simulink model "CRAB_TRACK"  (R2019b)
settings: Solver=VariableStepAuto  StartTime=0.0  StopTime=inf  RelTol=1e-3
undefined symbols (not defined in the file): Horn, magnitude, none, Rec, Schunck, SDTV, strel, videoinput
libraries: simulink x8, visionanalysis x3, visionconversions x2, visionstatistics x2, visionmorphops x2, dspsigattribs x2, dspindex x2, raspberrypilib x2, visiontextngfix x2, dspstat3 x2, imaqlib x1, dspmtrx3 x1
settings Model: Creator=danie  LastModifiedBy=danie

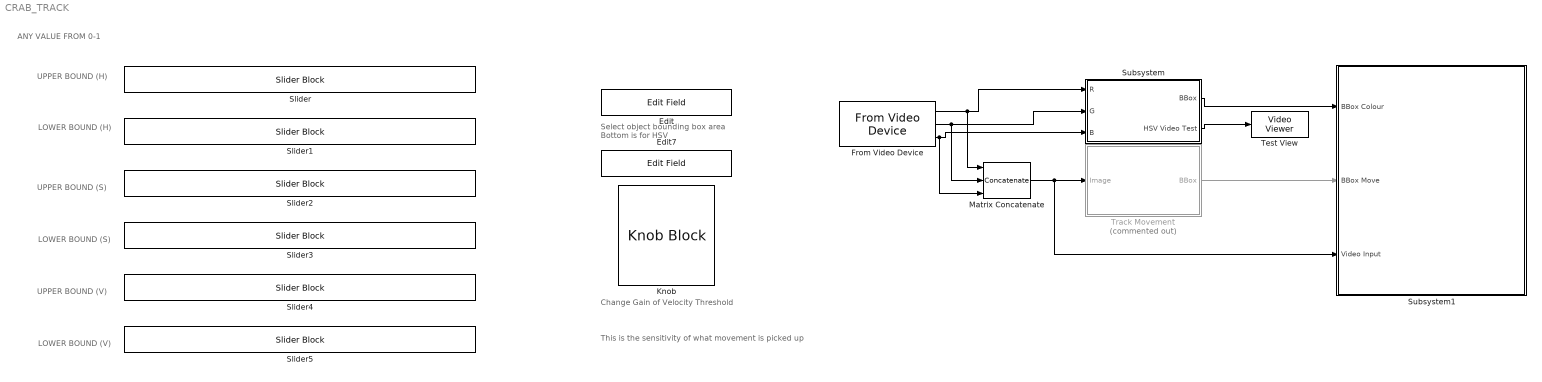
== system CRAB_TRACK ==
  note: ANY VALUE FROM 0-1
  note: LOWER BOUND (H)
  note: UPPER BOUND (H)
  note: This is the sensitivity of what movement is picked up
  note: Change Gain of Velocity Threshold
  note: Select object bounding box area
      | Bottom is for HSV
  note: UPPER BOUND (S)
  note: UPPER BOUND (V)
  note: LOWER BOUND (S)
  note: LOWER BOUND (V)
  Edit : EditField  LabelPosition=Hide  ShowInitialText=on  Alignment=Center
  Edit7 : EditField  LabelPosition=Hide  ShowInitialText=on  Alignment=Center
  From Video Device : imaqlib/From Video Device  DeviceMenu=winvideo 1 (USB_Camera)  Device=winvideo 1 (USB_Camera)  ObjConstructor=videoinput('winvideo', 1)  VideoFormatMenu=MJPG_1920x1080  VideoFormat=MJPG_1920x1080  VideoSource=input1  ROIPosition=[0 0 1080 1920]  EnableHWTrigger=off  TriggerConfiguration=none/none  SampleTime=1/30  OutputPortsMode=Separate color signals  DataType=single  CanDoHWTrigger=no  ReturnedColorSpace=rgb  BlockHandle=5428.0005  ROIWidth=1920  ROIHeight=1080  ROIColumn=0  ROIRow=0  EngXMLPath=E:\Matlab\toolbox\imaq\imaq\private  DevXMLPath=C:\ProgramData\MATLAB\SupportPackages\R2019b\toolbox\imaq\supportpackages\genericvideo\adaptor\win64  EngLibPath=E:\Matlab\toolbox\imaq\imaqblks\imaqmex\win64  ColorSpace=rgb  BayerSensorAlignment=grbg  ImaqMode=off
      settings: SourceProductName=Image Acquisition Toolbox
  Knob : KnobBlock
  Matrix Concatenate : Concatenate  NumInputs=3  Mode=Multidimensional array  ConcatenateDimension=3
  Slider{,1..5} (6 alike) : SliderBlock  ScaleMax=1
  Subsystem : Subsystem
  Subsystem1 : Subsystem
  Test View : VideoViewer  FigPos=[962 1037 958 929]
  Track Movement : Subsystem  Commented=on
  wires:
  From Video Device/1 -> Matrix Concatenate/1, Subsystem/1(R)
  Track Movement/1(BBox) -> Subsystem1/2(BBox Move)
  Subsystem/1(BBox) -> Subsystem1/1(BBox Colour)
  Subsystem/2(HSV Video Test) -> Test View/1
  From Video Device/2 -> Matrix Concatenate/2, Subsystem/2(G)
  From Video Device/3 -> Matrix Concatenate/3, Subsystem/3(B)
  Matrix Concatenate/1 -> Subsystem1/3(Video Input), Track Movement/1(Image)

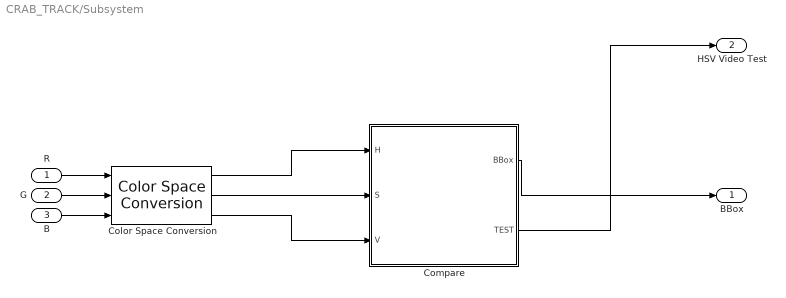
== system CRAB_TRACK/Subsystem ==
  R : Inport
  G : Inport  Port=2
  B : Inport  Port=3
  Color Space Conversion : visionconversions/Color Space  Conversion  conversion=Obsolete  conversionActive=R'G'B' to HSV  wp_str=D65  rec=Rec. 601 (SDTV)  sys=1125/60/2:1  imagePorts=Separate color signals
  Compare : Subsystem
  BBox : Outport
  HSV Video Test : Outport  Port=2
  wires:
  Compare/1(BBox) -> BBox/1
  Compare/2(TEST) -> HSV Video Test/1
  R/1 -> Color Space Conversion/1
  G/1 -> Color Space Conversion/2
  B/1 -> Color Space Conversion/3
  Color Space Conversion/1 -> Compare/1(H)
  Color Space Conversion/2 -> Compare/2(S)
  Color Space Conversion/3 -> Compare/3(V)

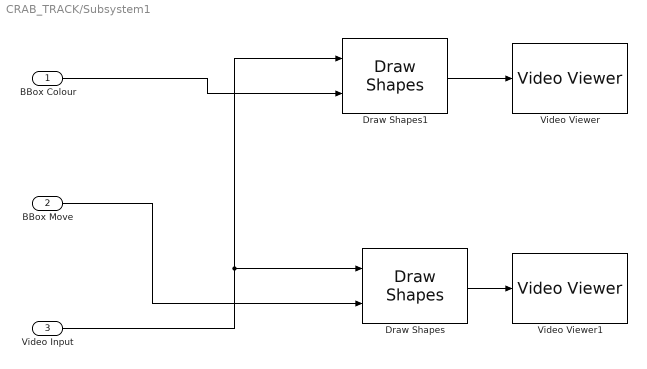
== system CRAB_TRACK/Subsystem1 ==
  BBox Colour : Inport
  BBox Move : Inport  Port=2
  Video Input : Inport  Port=3
  Draw Shapes : visiontextngfix/Draw Shapes  shape=Rectangles  fill=off  lineWidth=1  fillClrSource=Specify via dialog  display=User-specified value  intensity=200  color=[0 255 0]  opacity=0.6  viewport=Entire image  antialiasing=off  inType=Obsolete  imagePorts=One multidimensional signal  roundingMode=Floor  overflowMode=off  memoryMode=Specify word length  memoryWordLength=16  prodOutputMode=Binary point scaling  prodOutputWordLength=32  prodOutputFracLength=14  prodOutputSlope=2^-14  accumSlope=2^-14  memoryFracLength=15
      settings: SourceProductName=Computer Vision Toolbox
  Draw Shapes1 : visiontextngfix/Draw Shapes  shape=Rectangles  fill=off  lineWidth=1  fillClrSource=Specify via dialog  display=User-specified value  intensity=200  color=[0 255 0]  opacity=0.6  viewport=Entire image  antialiasing=off  inType=Obsolete  imagePorts=One multidimensional signal  roundingMode=Floor  overflowMode=off  memoryMode=Specify word length  memoryWordLength=16  prodOutputMode=Binary point scaling  prodOutputWordLength=32  prodOutputFracLength=14  prodOutputSlope=2^-14  accumSlope=2^-14  memoryFracLength=15
      settings: SourceProductName=Computer Vision Toolbox
  Video Viewer : VideoViewer  FigPos=[962 1037 958 929]
  Video Viewer1 : VideoViewer  FigPos=[2 517 958 409]
  wires:
  Draw Shapes/1 -> Video Viewer1/1
  Video Input/1 -> Draw Shapes1/1, Draw Shapes/1
  BBox Move/1 -> Draw Shapes/2
  Draw Shapes1/1 -> Video Viewer/1
  BBox Colour/1 -> Draw Shapes1/2

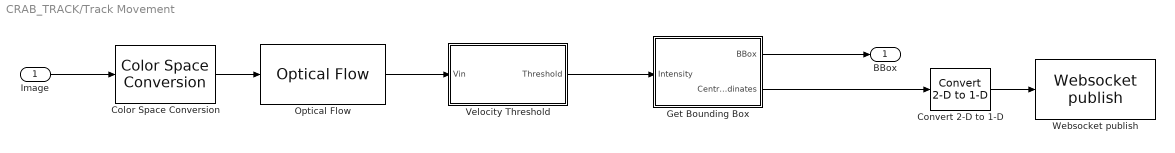
== system CRAB_TRACK/Track Movement ==
  Image : Inport
  Color Space Conversion : visionconversions/Color Space  Conversion  conversion=Obsolete  conversionActive=R'G'B' to intensity  wp_str=D65  rec=Rec. 601 (SDTV)  sys=1125/60/2:1  imagePorts=One multidimensional signal
  Convert 2-D to 1-D : dspsigattribs/Convert 2-D to 1-D
      settings: SourceProductName=DSP System Toolbox  SourceProductBaseCode=DS
  Get Bounding Box : Subsystem
  Optical Flow : visionanalysis/Optical Flow  method=Horn-Schunck  gradMethod=Difference filter [-1 1]  which2img=Current frame and N-th frame back  N=1  lambda=1  numInports=3  sigmaS=1.5  sigmaW=1  discardNormalFlow=off  outputCurrentImage=off  stop_criteria=When maximum number of iterations is reached  maxIter=10  maxAllowAbsDiff=eps  outVelForm=Horizontal and vertical components in complex form  eigTh=0.0039  roundingMode=Nearest  overflowMode=on  prodOutputMode=Binary point scaling  prodOutputWordLength=32  prodOutputFracLength=20  prodOutputSlope=2^-20  accumSlope=2^-20  memorySlope=2^-20  firstCoeffSlope=2^-20  outputMode=Binary point scaling  outputWordLength=32  outputFracLength=20  outputSlope=2^-20
      settings: SourceProductName=Computer Vision Toolbox  SourceProductBaseCode=VP
  Velocity Threshold : Subsystem
  Websocket publish : raspberrypilib/Websocket publish  UniqueBlockID=webPub 1  IPAddress=127.0.0.1  Port=9000  NumberOfSignals=1
      settings: SourceProductName=Simulink Support Package for Raspberry Pi Hardware  SourceProductBaseCode=RASPPI
  BBox : Outport
  wires:
  Image/1 -> Color Space Conversion/1
  Optical Flow/1 -> Velocity Threshold/1(Vin)
  Color Space Conversion/1 -> Optical Flow/1
  Velocity Threshold/1(Threshold) -> Get Bounding Box/1(Intensity)
  Get Bounding Box/2(Central Coordinates) -> Convert 2-D to 1-D/1
  Get Bounding Box/1(BBox) -> BBox/1
  Convert 2-D to 1-D/1 -> Websocket publish/1

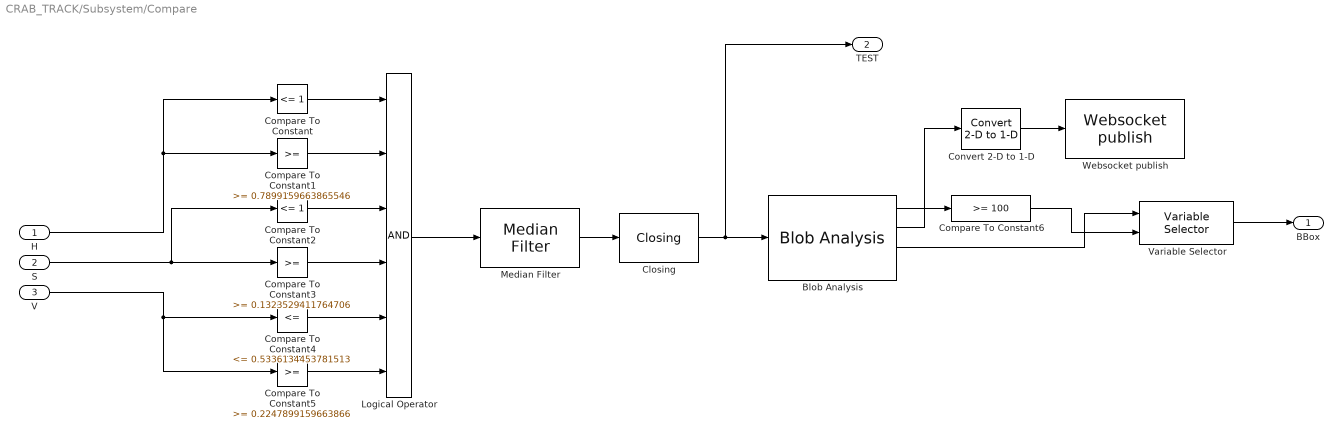
== system CRAB_TRACK/Subsystem/Compare ==
  H : Inport
  S : Inport  Port=2
  V : Inport  Port=3
  Blob Analysis : visionstatistics/Blob Analysis  Tag=vipblks_row_conv  area=on  centroid=on  bBox=on  majorAxis=off  minorAxis=off  angle=off  eccentricity=off  equivDiameterSq=off  extent=off  perimeter=off  outDT=double  conn=8  isLabel=on  maxBlobs=50  warnIfNumBlobsExceeded=on  isCount=off  useMinArea=off  minArea=0  useMaxArea=off  maxArea=intmax('uint32')  excludeBorderBlob=off  isOutVarDim=off  isFill=on  fillValues=-1  roundingMode=Floor  overflowMode=off  prodOutputMode=Binary point scaling  prodOutputWordLength=32  prodOutputFracLength=16  prodOutputSlope=2^-16  accumMode=Binary point scaling  accumWordLength=32  accumFracLength=0  accumSlope=2^0  outputMode=Binary point scaling  outputWordLength=32  outputFracLength=16  outputSlope=2^-16  memorySlope=2^-16  firstCoeffMode=Binary point scaling  firstCoeffWordLength=16  firstCoeffFracLength=14  firstCoeffSlope=2^-14  secondCoeffMode=Binary point scaling  secondCoeffWordLength=32  secondCoeffFracLength=16  secondCoeffSlope=2^-16
      settings: SourceProductName=Computer Vision Toolbox
  Closing : visionmorphops/Closing  nhoodsrc=Specify via dialog  strel=strel('line',5,45)
      settings: SourceProductName=Computer Vision Toolbox  SourceProductBaseCode=VP
  Compare To Constant : simulink/Logic and Bit Operations/Compare To Constant  relop=<=  const=1  OutDataTypeStr=boolean
  Compare To Constant1 : simulink/Logic and Bit Operations/Compare To Constant  relop=>=  const=0.7899159663865546  OutDataTypeStr=boolean
  Compare To Constant2 : simulink/Logic and Bit Operations/Compare To Constant  relop=<=  const=1  OutDataTypeStr=boolean
  Compare To Constant3 : simulink/Logic and Bit Operations/Compare To Constant  relop=>=  const=0.1323529411764706  OutDataTypeStr=boolean
  Compare To Constant4 : simulink/Logic and Bit Operations/Compare To Constant  relop=<=  const=0.5336134453781513  OutDataTypeStr=boolean
  Compare To Constant5 : simulink/Logic and Bit Operations/Compare To Constant  relop=>=  const=0.2247899159663866  OutDataTypeStr=boolean
  Compare To Constant6 : simulink/Logic and Bit Operations/Compare To Constant  relop=>=  const=100  OutDataTypeStr=boolean
  Convert 2-D to 1-D : dspsigattribs/Convert 2-D to 1-D
      settings: SourceProductName=DSP System Toolbox  SourceProductBaseCode=DS
  Logical Operator : Logic  Inputs=6  AllPortsSameDT=off  OutDataTypeStr=boolean
  Median Filter : visionanalysis/Median Filter  nghbood=[3 3]  outSize=Same as input port I  padType=Constant  padSrc=Specify via dialog  padVal=0  roundingMode=Floor  overflowMode=off  prodOutputSlope=2^-30  accumSlope=2^-30  outputSlope=2^-15
      settings: SourceProductName=Computer Vision Toolbox  SourceProductBaseCode=VP
  Variable Selector : dspindex/Variable Selector  NumInputs=1  rowsOrCols=Rows  IdxMode=Variable  Elements=[1 3]  ZerOneIdxMode=One-based  errmode=Clip Index  FillMode=on  FillValues=0
  Websocket publish : raspberrypilib/Websocket publish  UniqueBlockID=webPub 1  IPAddress=127.0.0.1  Port=9000  NumberOfSignals=1
      settings: SourceProductName=Simulink Support Package for Raspberry Pi Hardware  SourceProductBaseCode=RASPPI
  BBox : Outport
  TEST : Outport  Port=2
  wires:
  Compare To Constant/1 -> Logical Operator/1
  Compare To Constant1/1 -> Logical Operator/2
  Compare To Constant2/1 -> Logical Operator/3
  Compare To Constant3/1 -> Logical Operator/4
  Compare To Constant4/1 -> Logical Operator/5
  Compare To Constant5/1 -> Logical Operator/6
  Logical Operator/1 -> Median Filter/1
  H/1 -> Compare To Constant/1, Compare To Constant1/1
  S/1 -> Compare To Constant3/1, Compare To Constant2/1
  V/1 -> Compare To Constant5/1, Compare To Constant4/1
  Blob Analysis/2 -> Convert 2-D to 1-D/1
  Blob Analysis/3 -> Variable Selector/1
  Blob Analysis/1 -> Compare To Constant6/1
  Variable Selector/1 -> BBox/1
  Convert 2-D to 1-D/1 -> Websocket publish/1
  Compare To Constant6/1 -> Variable Selector/2
  Median Filter/1 -> Closing/1
  Closing/1 -> TEST/1, Blob Analysis/1

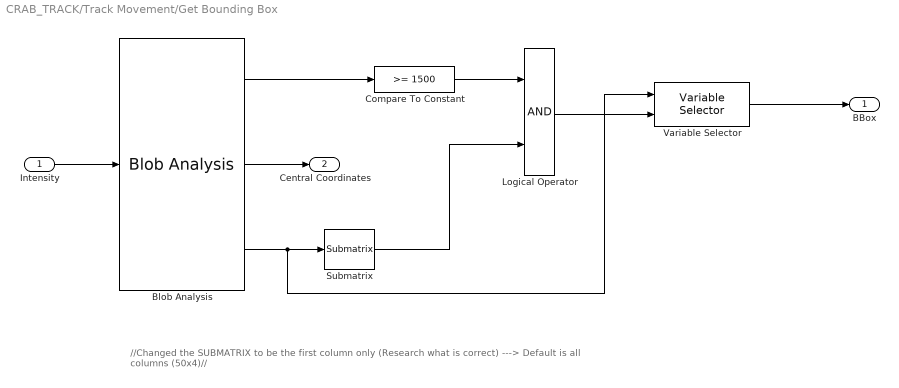
== system CRAB_TRACK/Track Movement/Get Bounding Box ==
  note: //Changed the SUBMATRIX to be the first column only (Research what is correct) ---> Default is all columns (50x4)//
  Intensity : Inport
  Blob Analysis : visionstatistics/Blob Analysis  Tag=vipblks_row_conv  area=on  centroid=on  bBox=on  majorAxis=off  minorAxis=off  angle=off  eccentricity=off  equivDiameterSq=off  extent=off  perimeter=off  outDT=double  conn=8  isLabel=off  maxBlobs=50  warnIfNumBlobsExceeded=on  isCount=off  useMinArea=off  minArea=0  useMaxArea=off  maxArea=intmax('uint32')  excludeBorderBlob=off  isOutVarDim=off  isFill=on  fillValues=-1  roundingMode=Floor  overflowMode=off  prodOutputMode=Binary point scaling  prodOutputWordLength=32  prodOutputFracLength=16  prodOutputSlope=2^-16  accumMode=Binary point scaling  accumWordLength=32  accumFracLength=0  accumSlope=2^0  outputMode=Binary point scaling  outputWordLength=32  outputFracLength=16  outputSlope=2^-16  memorySlope=2^-16  firstCoeffMode=Binary point scaling  firstCoeffWordLength=16  firstCoeffFracLength=14  firstCoeffSlope=2^-14  secondCoeffMode=Binary point scaling  secondCoeffWordLength=32  secondCoeffFracLength=16  secondCoeffSlope=2^-16
      settings: SourceProductName=Computer Vision Toolbox
  Compare To Constant : simulink/Logic and Bit Operations/Compare To Constant  relop=>=  const=1500  OutDataTypeStr=boolean
  Logical Operator : Logic  AllPortsSameDT=off  OutDataTypeStr=boolean
  Submatrix : dspmtrx3/Submatrix  RowSpan=All rows  RowStartMode=First  RowStartIndex=1  RowEndMode=Last  RowEndIndex=1  ColSpan=One column  ColStartMode=First  ColStartIndex=1  ColEndMode=Last  ColEndIndex=1
  Variable Selector : dspindex/Variable Selector  NumInputs=1  rowsOrCols=Rows  IdxMode=Variable  Elements=[1 3]  ZerOneIdxMode=One-based  errmode=Clip Index  FillMode=on  FillValues=0
  BBox : Outport
  Central Coordinates : Outport  Port=2
  wires:
  Intensity/1 -> Blob Analysis/1
  Blob Analysis/3 -> Variable Selector/1, Submatrix/1
  Compare To Constant/1 -> Logical Operator/1
  Submatrix/1 -> Logical Operator/2
  Logical Operator/1 -> Variable Selector/2
  Variable Selector/1 -> BBox/1
  Blob Analysis/2 -> Central Coordinates/1
  Blob Analysis/1 -> Compare To Constant/1

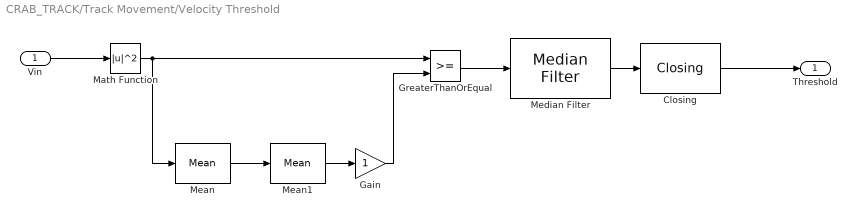
== system CRAB_TRACK/Track Movement/Velocity Threshold ==
  Vin : Inport
  Closing : visionmorphops/Closing  nhoodsrc=Specify via dialog  strel=strel('line',5,45)
      settings: SourceProductName=Computer Vision Toolbox  SourceProductBaseCode=VP
  Gain : Gain
  GreaterThanOrEqual : RelationalOperator  OutDataTypeStr=boolean  RndMeth=Simplest
  Math Function : Math  Operator=magnitude^2  SignedPower=off  SaturateOnIntegerOverflow=on
  Mean : dspstat3/Mean  run=off  InputProcessing=Columns as channels (frame based)  reset_popup=None  directionMode=Entire input  dimension=1  roiEnable=off  roiType=Rectangles  roiPortion=Entire ROI  roiOutput=Individual statistics for each ROI  roiFlag=off  roundingMode=Floor  overflowMode=off  outputDataTypeStr=Inherit: Same as accumulator  outputMin=[]  outputMax=[]  outputLastDataTypeStr=Inherit: Same as accumulator
  Mean1 : dspstat3/Mean  run=on  InputProcessing=Columns as channels (frame based)  reset_popup=None  directionMode=Each column  dimension=1  roiEnable=off  roiType=Rectangles  roiPortion=Entire ROI  roiOutput=Individual statistics for each ROI  roiFlag=off  roundingMode=Floor  overflowMode=off  outputDataTypeStr=Inherit: Same as accumulator  outputMin=[]  outputMax=[]  outputLastDataTypeStr=Inherit: Same as accumulator
  Median Filter : visionanalysis/Median Filter  nghbood=[3 3]  outSize=Same as input port I  padType=Constant  padSrc=Specify via dialog  padVal=0  roundingMode=Floor  overflowMode=off  prodOutputSlope=2^-30  accumSlope=2^-30  outputSlope=2^-15
      settings: SourceProductName=Computer Vision Toolbox  SourceProductBaseCode=VP
  Threshold : Outport
  wires:
  Vin/1 -> Math Function/1
  Math Function/1 -> Mean/1, GreaterThanOrEqual/1
  Mean/1 -> Mean1/1
  Mean1/1 -> Gain/1
  Gain/1 -> GreaterThanOrEqual/2
  GreaterThanOrEqual/1 -> Median Filter/1
  Median Filter/1 -> Closing/1
  Closing/1 -> Threshold/1
